simulink model "FTVsWBD_DoubleSupport"  (R2014a)
settings: Solver=FixedStepDiscrete  StartTime=0.0  StopTime=5  FixedStep=Ts  RelTol=1e-3
libraries: WBCLibrary x6
settings Model: Creator=jorhabib  LastModifiedBy=jorhabib

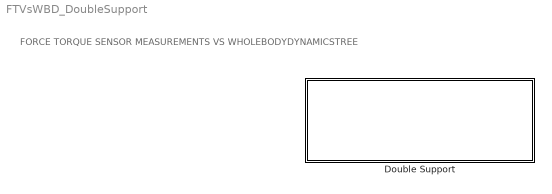
== system FTVsWBD_DoubleSupport ==
  note: FORCE TORQUE SENSOR MEASUREMENTS VS WHOLEBODYDYNAMICSTREE
  Double Support : Subsystem  mask{robotName='iCubGenova01', localName='simulink', Ts=0.010}
      mask prompts: robotName "Robot Name"; localName "Local Name"; Ts "Simulation Period"

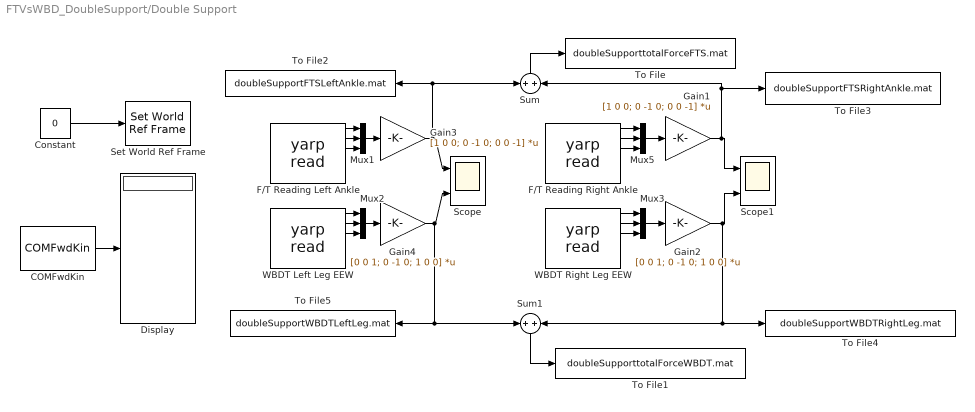
== system FTVsWBD_DoubleSupport/Double Support ==
  "COMFwdKin " : WBCLibrary/wholeBodyModel/Forward Kinematics/COMFwdKin   robotName=robotName  localName=localName
  Constant : Constant  Value=0  OutDataTypeStr=int8
  Display : Display
  F/T Reading Left Ankle : WBCLibrary/Utilities/yarp read  from=['/icub' '/left_foot/analog:o']  to='...'  num=6
  F/T Reading Right Ankle : WBCLibrary/Utilities/yarp read  from=['/icub' '/right_foot/analog:o']  to='...'  num=6
  Gain1 : Gain  Gain=[1 0 0; 0 -1 0; 0 0 -1]  Multiplication=Matrix(K*u)
  Gain2 : Gain  Gain=[0 0 1; 0 -1 0; 1 0 0]  Multiplication=Matrix(K*u)
  Gain3 : Gain  Gain=[1 0 0; 0 -1 0; 0 0 -1]  Multiplication=Matrix(K*u)
  Gain4 : Gain  Gain=[0 0 1; 0 -1 0; 1 0 0]  Multiplication=Matrix(K*u)
  Mux{1..3,5} (4 alike) : Mux  Inputs=3
  Scope : Scope  NumInputPorts=2
      settings: YMin=-20~-25  YMax=180~175
  Scope1 : Scope  NumInputPorts=2
      settings: YMin=40~-30  YMax=130~140
  Set World Ref Frame : WBCLibrary/wholeBodyModel/Set World Ref Frame  robotName=robotName  localName=localName
  Sum : Sum
  Sum1 : Sum
  To File : ToFile  Filename=doubleSupporttotalForceFTS.mat  MatrixName=doubleSupporttotalForceFTS  SaveFormat=Timeseries
  To File1 : ToFile  Filename=doubleSupporttotalForceWBDT.mat  MatrixName=doubleSupporttotalForceWBDT  SaveFormat=Timeseries
  To File2 : ToFile  Filename=doubleSupportFTSLeftAnkle.mat  MatrixName=doubleSupportFTSLeftAnkle  SaveFormat=Timeseries
  To File3 : ToFile  Filename=doubleSupportFTSRightAnkle.mat  MatrixName=doubleSupportFTSRightAnkle  SaveFormat=Timeseries
  To File4 : ToFile  Filename=doubleSupportWBDTRightLeg.mat  MatrixName=doubleSupportWBDTRightLeg  SaveFormat=Timeseries
  To File5 : ToFile  Filename=doubleSupportWBDTLeftLeg.mat  MatrixName=doubleSupportWBDTLeftLeg  SaveFormat=Timeseries
  WBDT Left Leg EEW : WBCLibrary/Utilities/yarp read  from=['/wholeBodyDynamicsTree' '/left_leg/endEffectorWrench:o']  to='...'  num=6
  WBDT Right Leg EEW : WBCLibrary/Utilities/yarp read  from=['/wholeBodyDynamicsTree' '/right_leg/endEffectorWrench:o']  to='...'  num=6
  wires:
  "COMFwdKin "/1 -> Display/1
  Constant/1 -> Set World Ref Frame/1
  WBDT Left Leg EEW/2 -> Mux2/2
  WBDT Left Leg EEW/1 -> Mux2/1
  WBDT Left Leg EEW/3 -> Mux2/3
  Gain4/1 -> To File5/1, Sum1/1, Scope/2
  Gain3/1 -> To File2/1, Sum/1, Scope/1
  Gain1/1 -> Sum/2, To File3/1, Scope1/1
  Gain2/1 -> To File4/1, Sum1/2, Scope1/2
  F/T Reading Left Ankle/1 -> Mux1/1
  F/T Reading Left Ankle/2 -> Mux1/2
  F/T Reading Left Ankle/3 -> Mux1/3
  Mux1/1 -> Gain3/1
  Mux2/1 -> Gain4/1
  F/T Reading Right Ankle/1 -> Mux5/1
  F/T Reading Right Ankle/2 -> Mux5/2
  F/T Reading Right Ankle/3 -> Mux5/3
  WBDT Right Leg EEW/1 -> Mux3/1
  WBDT Right Leg EEW/2 -> Mux3/2
  WBDT Right Leg EEW/3 -> Mux3/3
  Mux5/1 -> Gain1/1
  Mux3/1 -> Gain2/1
  Sum/1 -> To File/1
  Sum1/1 -> To File1/1
